simulink model "Steuerung"  (R2018a)
settings: Solver=ode1  StartTime=0.0  StopTime=inf  FixedStep=1/10  RelTol=1e-3  EnableMultiTasking=on
undefined symbols (not defined in the file or in its folder): gray, Rows
libraries: PiCar_library x4, simulink x3, dspsigops x1
settings Model: SimulationMode=external  Creator=raspberry  LastModifiedBy=timha
settings SolverCC: PositivePriorityOrder=on
settings OptimizationCC: PassReuseOutputArgsAs=Individual arguments  MaxStackSize=64
settings DebuggingCC: ParameterTunabilityLossMsg=error
settings HardwareCC: ProdBitPerPointer=32  ProdBitPerSizeT=32  ProdBitPerPtrDiffT=32  ProdLargestAtomicInteger=Long  ProdLargestAtomicFloat=Double  ProdWordSize=32  ProdHWDeviceType=ARM Compatible->ARM Cortex
settings SFSimCC: MATLABDynamicMemAlloc=off
settings RTWCC: SystemTargetFile=ert.tlc  HardwareBoard=Raspberry Pi  TLCOptions="-aInlineSetEventsForThisBaseRateFcn=TLC_FALSE -aSuppressMultiTaskScheduler=TLC_FALSE  -aRateBasedStepFcn=0"  TemplateMakefile=ert_default_tmf  Toolchain=GNU GCC Raspberry Pi
settings RTWCC: CustomTerminator=|
  | /* Send ALL_LED_OFF Signal to all PWM driver chip address
  | See PCA9685 user manual, section 7.3.4
  | Set Chip in sleep mode, section 7.3.1
  | Reset the PWM ON/OFF states for all LEDs */
  | 
  | int fd;
  | 
  | fd = wiringPiI2CSetup(0x70);
  | wiringPiI2CWriteReg8(fd, 0x00, 0x11); // sleep mode
  | wiringPiI2CWriteReg8(fd, 0xFD, 0x10); // all LED off
  | wiringPiI2CWriteReg8(fd, 0xFC, 0x00);
  | wiringPiI2CWriteReg8(fd, 0xFB, 0x00);
  | wiringPiI2CWriteReg8(fd, 0xFA, 0x00);
settings CodeAppCC: ForceParamTrailComments=on  IgnoreCustomStorageClasses=off  OperatorAnnotations=on  SimulinkDataObjDesc=on  SFDataObjDesc=on  MATLABFcnDesc=on  InsertBlockDesc=on  StateflowObjectComments=on  MATLABSourceComments=on
settings ERTTargetCC: SupportVariableSizeSignals=on

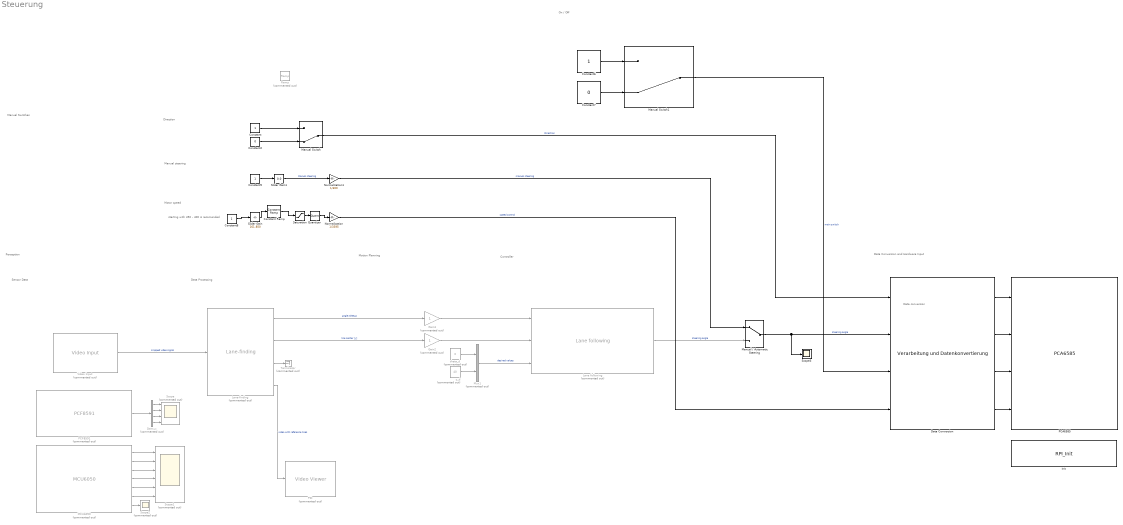
== system Steuerung ==
  note: starting with 350 - 400 is recomended
  note: Data Conversion and Hardware Input
  note: Data conversion
  note: Manual Switches
  note: Motion Planning
  note: Perception
  note: Controller
  note: Data Processing
  note: Sensor Data
  note: Manual steering
  note: Motor speed
  note: Direction
  note: On / Off
  Constant{,5..6,8} (4 alike) : Constant
  Constant Ramp : dspsigops/Constant Ramp  L=Rows  dim=1  Slope=20  dataType=Same as input  isSigned=on  wordLen=16  udDataType=sfix(16)  fracBitsMode=Best precision  numFracBits=15  Offset=0
      settings: SourceProductName=DSP System Toolbox  SourceProductBaseCode=DS
  Constant2 : Constant  Value=0
  Constant7 : Constant  Value=0
  Data Conversion : PiCar_library/Verarbeitung und Datenkonvertierung
      link override Constant3: Value=1180
  Demux : Demux  Commented=on
  Gain2 : Gain  Commented=on
  Gain3 : Gain  Commented=on
  Init : S-Function  Priority=1  InitFcn=try, set_param(gcb,'FunctionName','RPI_Init'), end  FunctionName=RPI_Init  SFunctionModules=RPI_Init_wrapper  SFunctionDeploymentMode=off  EnableBusSupport=off  mask(S-Function Builder){}
      mask help: Simulink:masks:SFunctionBuilder_MD
      mask init:
      | val = [[.9  0.75 0.75 1 1 .9 .9 1]',[1 1 0.75 0.75 .9 .9 1 .9]'];try , sys = get_param(gcb,'SfunBuilderFcnName');if isempty(sys), sys = get_param(gcb,'FunctionName'); end,catch, sys = get_param(gcb,'FunctionName'); end
      settings: CopyFcn=set_param(gcbh,'LinkStatus','none')  PreSaveFcn=try, set_param(gcb,'FunctionName','RPI_Init'), end  OpenFcn=sfunctionwizard(gcbh)
      mask Display:
      | plot(val(:,1),val(:,2))
      | disp(sys)
  Lane following : PiCar_library/Lane following  Commented=on
  Lane-finding : PiCar_library/Lane-finding  Commented=on
  MCU6050 : S-Function  Commented=on  InitFcn=try, set_param(gcb,'FunctionName','MCU6050'), end  FunctionName=MCU6050  SFunctionModules=MCU6050_wrapper  SFunctionDeploymentMode=off  EnableBusSupport=off  mask(S-Function Builder){}
      mask help: Simulink:masks:SFunctionBuilder_MD
      mask init: same as Steuerung/Init
      settings: CopyFcn=set_param(gcbh,'LinkStatus','none')  PreSaveFcn=try, set_param(gcb,'FunctionName','MCU6050'), end  OpenFcn=sfunctionwizard(gcbh)
      mask Display: plot(val(:,1),val(:,2)),disp(sys), port_label('output',1,'ax'), port_label('output',2,'ay'), port_label('output',3,'az'), port_label('output',4,'omx'), port_label('output',5,'omy'), port_label('output',6,'omz'), port_label('output',7,'temp')
  Manual / Automatic Steering : ManualSwitch
  Manual Switch : ManualSwitch  CurrentSetting=0
  Manual Switch1 : ManualSwitch  CurrentSetting=0
  Mux1 : Mux  Commented=on  Inputs=2
  Normalization : Gain  Gain=1/3395
  Normalization1 : Gain  Gain=1/300
  PCA6585 : S-Function  InitFcn=try, set_param(gcb,'FunctionName','PCA6585'), end  FunctionName=PCA6585  SFunctionModules=PCA6585_wrapper  SFunctionDeploymentMode=off  EnableBusSupport=off  mask(S-Function Builder){}
      mask help: Simulink:masks:SFunctionBuilder_MD
      mask init: same as Steuerung/Init
      settings: CopyFcn=set_param(gcbh,'LinkStatus','none')  PreSaveFcn=try, set_param(gcb,'FunctionName','PCA6585'), end  OpenFcn=sfunctionwizard(gcbh)
      mask Display: plot(val(:,1),val(:,2)),disp(sys), port_label('input',1,'IN_1'), port_label('input',2,'IN_2'), port_label('input',3,'PWM'), port_label('input',4,'SERVO')
  PCF8591 : S-Function  Commented=on  InitFcn=try, set_param(gcb,'FunctionName','PCF8591'), end  FunctionName=PCF8591  SFunctionModules=PCF8591_wrapper  SFunctionDeploymentMode=off  EnableBusSupport=off  mask(S-Function Builder){}
      mask help: Simulink:masks:SFunctionBuilder_MD
      mask init: same as Steuerung/Init
      settings: CopyFcn=set_param(gcbh,'LinkStatus','none')  PreSaveFcn=try, set_param(gcb,'FunctionName','PCF8591'), end  OpenFcn=sfunctionwizard(gcbh)
      mask Display: plot(val(:,1),val(:,2)),disp(sys), port_label('output',1,'PCF8591_out')
  PID : VideoViewer  Commented=on  colormapValue=gray(256)  FigPos=[887.285714285714 806 554.857142857143 305.714285714286]
  Quantizer : Quantizer  QuantizationInterval=1
  Ramp : simulink/Sources/Ramp  Commented=on  slope=1  start=0  InitialOutput=0
  Saturation : Saturate  UpperLimit=3000
  Scope : Scope  Commented=on  NumInputPorts=4
  Scope1 : Scope  Commented=on  NumInputPorts=6
  Scope2 : Scope  Commented=on
  Scope3 : Scope
  Slider Gain : simulink/Math Operations/Slider Gain  gain=161.850  low=0  high=5395
  Slider Gain1 : simulink/Math Operations/Slider Gain  gain=0.0  low=-300  high=300
  Terminator : Terminator  Commented=on
  Video Input : PiCar_library/Video Input  Commented=on
  theta_d : Constant  Commented=on  Value=0
  y_d : Constant  Commented=on  Value=40
  wires:
  Constant/1 -> Manual Switch/1
  Constant2/1 -> Manual Switch/2
  Constant7/1 -> Manual Switch1/2
  Constant6/1 -> Manual Switch1/1
  Slider Gain1/1 -> Normalization1/1  "Manual steering"
  Lane-finding/2 -> Gain2/1  "line center [y]"
  Demux/3 -> Scope/3
  Demux/4 -> Scope/4
  PCF8591/1 -> Demux/1
  MCU6050/2 -> Scope1/2
  MCU6050/3 -> Scope1/3
  MCU6050/1 -> Scope1/1
  MCU6050/4 -> Scope1/4
  MCU6050/5 -> Scope1/5
  MCU6050/6 -> Scope1/6
  MCU6050/7 -> Scope2/1
  Manual Switch/1 -> Data Conversion/1  "Direction"
  Manual / Automatic Steering/1 -> Data Conversion/2, Scope3/1  "steering angle"
  Manual Switch1/1 -> Data Conversion/3  "main switch"
  Data Conversion/1 -> PCA6585/1
  Data Conversion/2 -> PCA6585/2
  Data Conversion/3 -> PCA6585/3
  Data Conversion/4 -> PCA6585/4
  Video Input/1 -> Lane-finding/1  "cropped video signal"
  Lane-finding/1 -> Gain3/1  "angle [theta]"
  Lane following/1 -> Manual / Automatic Steering/2  "steering angle"
  Slider Gain/1 -> Constant Ramp/1
  Lane-finding/3 -> Terminator/1
  Lane-finding/4 -> PID/1  "video with reference lines"
  Normalization/1 -> Data Conversion/4  "speed control"
  y_d/1 -> Mux1/2
  theta_d/1 -> Mux1/1
  Mux1/1 -> Lane following/3  "desired values"
  Normalization1/1 -> Manual / Automatic Steering/1  "manual steering"
  Demux/1 -> Scope/1
  Demux/2 -> Scope/2
  Gain3/1 -> Lane following/1
  Gain2/1 -> Lane following/2
  Quantizer/1 -> Normalization/1
  Constant8/1 -> Slider Gain/1
  Constant5/1 -> Slider Gain1/1
  Constant Ramp/1 -> Saturation/1
  Saturation/1 -> Quantizer/1
